simulink model "Sim"  (R2024b)
settings: Solver=VariableStepAuto  StartTime=0.0  StopTime=20  RelTol=1e-3
values from neighbouring files (symbols this model uses):
  hiddenLayerSize = 2 * inputLayerSize + 1    (= 7)    [Init.m]
  inputLayerSize = n + 1    (= 3)    [Init.m]
  outputLayerSize = 2    [Init.m]
settings Model: Creator=Asus  LastModifiedBy=Asus

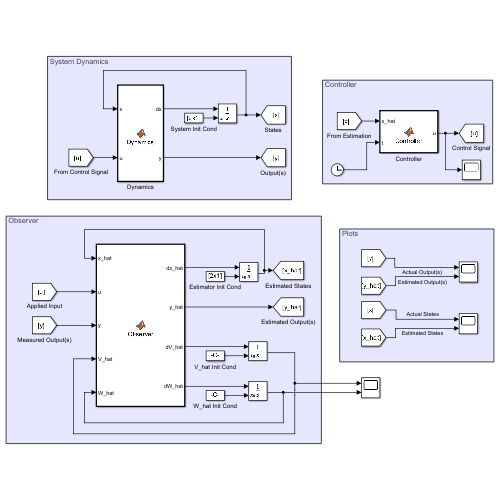
[thumbnail: Simulink's stored preview of the top-level diagram]
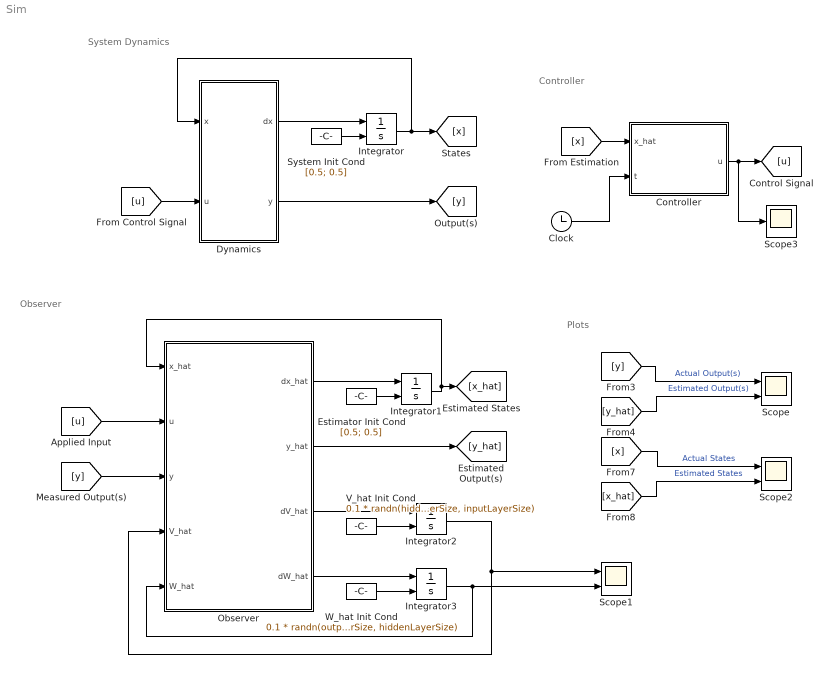
== system Sim ==
  note: Controller
  note: Plots
  note: System Dynamics
  note: Observer
  Clock : Clock
  Controller : MATLAB Function  TreatAsAtomicUnit=on
  Dynamics : MATLAB Function  TreatAsAtomicUnit=on
  Estimator Init Cond : Constant  Value=[0.5; 0.5]
  Integrator : Integrator  InitialConditionSource=external  InitialCondition=[0.5; 0.5]
  Integrator1 : Integrator  InitialConditionSource=external  InitialCondition=[0.5; 0.5]
  Integrator2 : Integrator  InitialConditionSource=external  InitialCondition=0.1 * randn(hiddenLayerSize, inputLayerSize)
  Integrator3 : Integrator  InitialConditionSource=external  InitialCondition=0.1 * randn(outputLayerSize, hiddenLayerSize)
  Observer : MATLAB Function  TreatAsAtomicUnit=on
  Scope : Scope  NumInputPorts=2
  Scope1 : Scope  NumInputPorts=2
  Scope2 : Scope  NumInputPorts=2
  Scope3 : Scope
  System Init Cond : Constant  Value=[0.5; 0.5]
  V_hat Init Cond : Constant  Value=0.1 * randn(hiddenLayerSize, inputLayerSize)
  W_hat Init Cond : Constant  Value=0.1 * randn(outputLayerSize, hiddenLayerSize)
  wires:
  Observer/3(dV_hat) -> Integrator2/1
  Integrator1/1 -> Observer/1(x_hat), [x_hat]
  Estimator Init Cond/1 -> Integrator1/2
  Observer/1(dx_hat) -> Integrator1/1
  Integrator3/1 -> Scope1/2, Observer/5(W_hat)
  [x] -> Scope2/1  "Actual States"
  [x_hat] -> Scope2/2  "Estimated States"
  Dynamics/2(y) -> [y]
  W_hat Init Cond/1 -> Integrator3/2
  Integrator2/1 -> Scope1/1, Observer/4(V_hat)
  Dynamics/1(dx) -> Integrator/1
  Controller/1(u) -> [u], Scope3/1
  [y] -> Scope/1  "Actual Output(s)"
  System Init Cond/1 -> Integrator/2
  V_hat Init Cond/1 -> Integrator2/2
  [u] -> Dynamics/2(u)
  [y] -> Observer/3(y)
  Integrator/1 -> [x], Dynamics/1(x)
  [y_hat] -> Scope/2  "Estimated Output(s)"
  Observer/4(dW_hat) -> Integrator3/1
  Observer/2(y_hat) -> [y_hat]
  [x] -> Controller/1(x_hat)
  [u] -> Observer/2(u)
  Clock/1 -> Controller/2(t)

== matlab function Sim/Controller ==
  data: u output; x_hat input; t input
function u = Controller(x_hat, t)
    
    u = - [3, 5] * (x_hat - [sin(t); cos(t)]); % simple observer-based state feedback

end

== matlab function Sim/Dynamics ==
  data: x input; dx output; y output; u input
function [dx, y] = Dynamics(x, u)

    fx  = [x(2); x(2) - x(1)];
    gx  = [0; 1];               
    C   = [1, 0];               

    dx  = fx + gx * u;
    y   = C * x;

end

== matlab function Sim/Observer ==
  data: dx_hat output; x_hat input; u input; y_hat output; y input; V_hat input; W_hat input; dV_hat output; dW_hat output
function [dx_hat, y_hat, dV_hat, dW_hat] = Observer(x_hat, u, y, V_hat, W_hat)
    
    % arbitrary hurwitz matrix
    A = [0, 1; -1, -2];

    % system output matrix
    C = [1, 0];

    % observer gain
    % G = [-19, 7]';
    G = [1, 1]';

    % closed loop state matrix
    Ac = A - G * C;

    % designing params
    eta = 1 * [70; 70];
    rho = 1 * [0.1; 0.1];

    % hidden layer activation function
    kernel = @(z) (-1 + 2 ./ (1 + exp(-2 * z)));

    % neural network input
    xNN = [x_hat; u];

    % estimation of nonlinear terms
    g_hat  = W_hat * kernel(V_hat * xNN);
 
    % observer model
    dx_hat = A * x_hat + g_hat + G * (y - C * x_hat);
    y_hat  = C * x_hat;

    % observer error
    y_tilde = y - y_hat;

    % output layer weights adaption law
    dW_hat = - eta(1) * ((y_tilde' * C * inv(Ac) * ones(size(Ac, 1), 1))' * kernel(V_hat * xNN) - rho(1) * sqrt(y_tilde' * y_tilde) * W_hat')'; %#ok
    % dW_hat = zeros(size(W_hat));

    % input layer weights adaption law
    dV_hat = - eta(2) * (y_tilde' * C * inv(Ac) * W_hat * (eye(size(W_hat, 2)) - diag((kernel(V_hat * xNN)).^2)))' * xNN' - ...
        rho(2) * sqrt(y_tilde' * y_tilde) * V_hat; %#ok
    % dV_hat = zeros(size(V_hat));

end
